simulink library "pwrsysBasic"  (R2016a)
settings: Solver=VariableStepAuto  SolverMode=SingleTasking  StartTime=0.0  StopTime=10.0  RelTol=1e-3
values from neighbouring files (symbols this model uses):
  Ts = Ts_c    (= 1e-07)    [PlantStateEquations_abc_Script.m]
undefined symbols (not defined in the file or in its folder): DiscIntNeverNeededParam, fn, Iap, Uanp
undefined symbols (not defined in the file): Sn, tctrl
libraries: pwrsysBasic x15, powerlib_meascontrol x12, pwrsysTransf x8, simulink x2
(part 2 of 2)

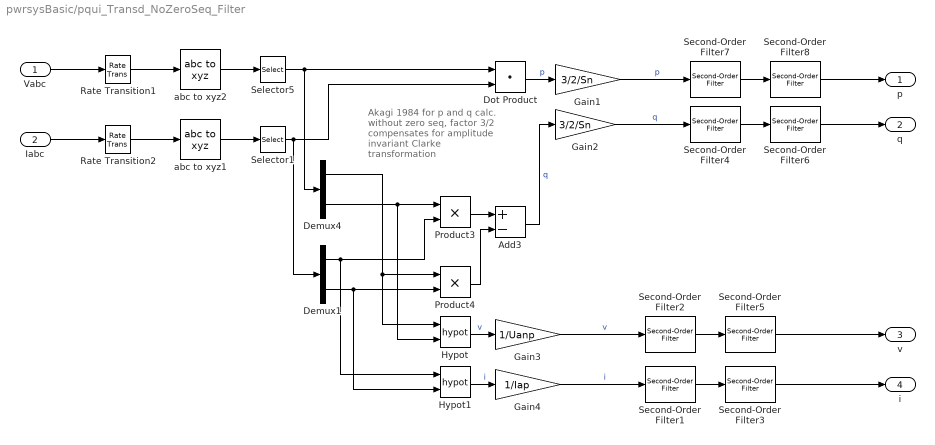
== system pwrsysBasic/pqui_Transd_NoZeroSeq_Filter ==
  note: Akagi 1984 for p and q
      | calc. without zero seq,
      | factor 3/2 compensates for
      | amplitude invariant
      | Clarke transformation
  Vabc : Inport
  Iabc : Inport  Port=2
  Add3 : Sum  Inputs=+-
  Demux1 : Demux  Outputs=2
  Demux4 : Demux  Outputs=2
  Dot Product : DotProduct  InputSameDT=on  OutDataTypeStr=Inherit: Inherit via internal rule
  Gain1 : Gain  Gain=3/2/Sn
  Gain2 : Gain  Gain=3/2/Sn
  Gain3 : Gain  Gain=1/Uanp
  Gain4 : Gain  Gain=1/Iap
  Hypot : Math  Operator=hypot  RndMeth=Zero  SaturateOnIntegerOverflow=on
  Hypot1 : Math  Operator=hypot  RndMeth=Zero  SaturateOnIntegerOverflow=on
  Product3 : Product
  Product4 : Product
  Rate Transition1 : RateTransition  OutPortSampleTime=Ts
  Rate Transition2 : RateTransition  OutPortSampleTime=Ts
  Second-Order Filter1 : powerlib_meascontrol/Filters/Second-Order Filter  FilterType=Lowpass  Fo=fcutoutvi  Zeta=zeta  Ts=Ts  Initialize=off  Vac_Init="[0,  0,  60]"  Vdc_Init=0  PlotResponse=off  FreqRange=[0, 1000, 0.1]
  Second-Order Filter2 : powerlib_meascontrol/Filters/Second-Order Filter  FilterType=Lowpass  Fo=fcutoutvi  Zeta=zeta  Ts=Ts  Initialize=off  Vac_Init="[0,  0,  60]"  Vdc_Init=0  PlotResponse=off  FreqRange=[0, 1000, 0.1]
  Second-Order Filter{3,5..6,8} (4 alike) : powerlib_meascontrol/Filters/Second-Order Filter  FilterType=Bandstop (Notch)  Fo=fn  Zeta=zeta  Ts=Ts  Initialize=off  Vac_Init="[0,  0,  60]"  Vdc_Init=0  PlotResponse=off  FreqRange=[0, 1000, 0.1]
  Second-Order Filter4 : powerlib_meascontrol/Filters/Second-Order Filter  FilterType=Lowpass  Fo=fcutoutpq  Zeta=zeta  Ts=Ts  Initialize=off  Vac_Init="[0,  0,  60]"  Vdc_Init=0  PlotResponse=off  FreqRange=[0, 1000, 0.1]
  Second-Order Filter7 : powerlib_meascontrol/Filters/Second-Order Filter  FilterType=Lowpass  Fo=fcutoutpq  Zeta=zeta  Ts=Ts  Initialize=off  Vac_Init="[0,  0,  60]"  Vdc_Init=0  PlotResponse=off  FreqRange=[0, 1000, 0.1]
  Selector1 : Selector  InputPortWidth=3  IndexOptions=Index vector (dialog)  Indices=[1 2]  OutputSizes=1
  Selector5 : Selector  InputPortWidth=3  IndexOptions=Index vector (dialog)  Indices=[1 2]  OutputSizes=1
  abc to xyz1 : pwrsysTransf/abc to xyz  typeTransf=Amplitude-invariant
  abc to xyz2 : pwrsysTransf/abc to xyz  typeTransf=Amplitude-invariant
  p : Outport
  q : Outport  Port=2
  v : Outport  Port=3
  i : Outport  Port=4
  wires:
  abc to xyz1/1 -> Selector1/1
  Gain3/1 -> Second-Order Filter2/1  "v"
  Demux1/2 -> Hypot1/2, Product4/2
  Hypot1/1 -> Gain4/1  "i"
  Selector1/1 -> Demux1/1, Dot Product/2
  Selector5/1 -> Demux4/1, Dot Product/1
  Demux4/1 -> Hypot/1, Product4/1
  Hypot/1 -> Gain3/1  "v"
  Iabc/1 -> Rate Transition2/1
  Dot Product/1 -> Gain1/1  "p"
  Demux1/1 -> Hypot1/1, Product3/2
  Add3/1 -> Gain2/1  "q"
  Vabc/1 -> Rate Transition1/1
  Product4/1 -> Add3/2
  Demux4/2 -> Hypot/2, Product3/1
  Rate Transition1/1 -> abc to xyz2/1
  abc to xyz2/1 -> Selector5/1
  Rate Transition2/1 -> abc to xyz1/1
  Product3/1 -> Add3/1
  Gain1/1 -> Second-Order Filter7/1  "p"
  Gain4/1 -> Second-Order Filter1/1  "i"
  Gain2/1 -> Second-Order Filter4/1  "q"
  Second-Order Filter2/1 -> Second-Order Filter5/1
  Second-Order Filter5/1 -> v/1
  Second-Order Filter1/1 -> Second-Order Filter3/1
  Second-Order Filter3/1 -> i/1
  Second-Order Filter4/1 -> Second-Order Filter6/1
  Second-Order Filter6/1 -> q/1
  Second-Order Filter8/1 -> p/1
  Second-Order Filter7/1 -> Second-Order Filter8/1

== system pwrsysBasic/var_delay_floor_ceiling ==
  x(k) : Inport
  n : Inport  Port=2
  S-Function : S-Function  FunctionName=variable_delay_floor_ceil  Parameters=200  SFunctionDeploymentMode=off  EnableBusSupport=off
  x(k-nf) : Outport
  x(k-nc) : Outport  Port=2
  wires:
  n/1 -> S-Function/2
  x(k)/1 -> S-Function/1
  S-Function/1 -> x(k-nf)/1
  S-Function/2 -> x(k-nc)/1

== matlab function pwrsysBasic/digital_ramp_gen/MATLAB Function ==
  data: up input; down input; rate input; y output; max input; min input; force input; forceval input; Ts input
%%%%%%%%%%%%%%%%%%%%%%%%%%%%%%%%%%%%%%%%%%%%%%%%%%%%%%%%%%%%%%%%%%%%%%%%%%
% Digital integrator
%%%%%%%%%%%%%%%%%%%%%%%%%%%%%%%%%%%%%%%%%%%%%%%%%%%%%%%%%%%%%%%%%%%%%%%%%%\
% Forward Euler method: as in matlab help
%   y(n) = y(n-1) + Ts(n-1)*x(n-1)
%   uset it to avoid algebraic loops

% All inputs are stored in states, so there is no direct feedthrough
% GAMBIARRA for avoiding algebraic loops
% see: https://www.mathworks.com/help/simulink/ug/integration-considerations-for-matlab-function-blocks.html

% Inputs
%   up: ramps up
%   down: ramps down (if both up and down, than stops)
%   max: max value for ramp
%   min: min value for ramp
%   force: if=1 sets integrator to forceval
%   forceval: see line above (max and min are respected
%   Ts: sampling time
% Output
%   y: output of the ramp

%%%%%%%%%%%%%%%%%%%%%%%%%%%%%%%%%%%%%%%%%%%%%%%%%%%%%%%%%%%%%%%%%%%%%%%%%%\
% Prog/rev history
%   Mota - 2021-05-21: first release

function y = DigRamp(up, down, rate, max, min, force, forceval, Ts)

% The value of the integrator
persistent i
persistent old_up
persistent old_down
persistent old_rate
persistent old_max
persistent old_min
persistent old_force
persistent old_forceval
persistent old_Ts

% Only at first cycle - outputs zero
if isempty(i)
    y = 0;
    i = 0;
    old_up = 0;
    old_down = 0;
    old_rate = 0;
    old_max = 0;
    old_min = 0;
    old_force = 0;
    old_forceval = 0;
    old_Ts = 0;
    % On the second cycle, output will still be zero, due to choices above
    return;
end

% auxiliary value
aux = 0;

% Bypassing the integrator with a value (can be used for followup)
if old_force == 1
    aux = old_forceval;
else
    %if not bypass, then calculate the next value of the integrator
    aux = i + old_Ts*old_rate*old_up + old_Ts*old_rate*old_down ;
end

%Limiting the integrator
if aux > old_max
    % max value has priority, i.e.,
    % if "max" is below "min" due to engineer error
    % the integrator will stop at "max"
    aux = old_max;
elseif aux < old_min
    % if integrator would cross the min, it will be stopped at min
    aux = old_min;
end

% output of the integrator
y = aux;

%update states
i = aux;
old_rate = rate;
%ramps up if up > 0
if up > 0
    old_up = 1;
else
    old_up = 0;
end
%ramps down if down > 0
if down > 0 
    old_down = -1;
else
    old_down = 0;
end
old_max = max;
old_min = min;
old_force = force;
old_forceval = forceval;
old_Ts = Ts;
